simulink model "Channelizer_demo"  (R2023b)
settings: Solver=VariableStepAuto  StartTime=0.0  StopTime=inf  RelTol=1e-3
PostLoadFcn:
  | TT = numerictype(1,16,15);
  | FF = fimath('RoundingMethod','Nearest','OverflowAction','Saturate');
  | mdl = channelizer_init(TT, FF);
  | channelizer = channelizer_model(mdl, TT, FF );
  | Ts = 16*(7/4)/8.75e9;
  | ch_filt_coef = rcosdesign(0.22,4,28,'normal');
  | ch_filt_coef = 28 * ch_filt_coef / sum(ch_filt_coef(:));
  | channelizer_demo_init;
values from neighbouring files (symbols this model uses):
  ch0_en = 0    [channelizer_demo_init.m]    (also in init.m)
  ch0_qam = 0    [channelizer_demo_init.m]    (also in init.m)
  ch0_swp = 0    [channelizer_demo_init.m]    (also in init.m)
  ch10_en = 0    [channelizer_demo_init.m]    (also in init.m)
  ch10_qam = 0    [channelizer_demo_init.m]    (also in init.m)
  ch10_swp = 0    [channelizer_demo_init.m]    (also in init.m)
  ch11_en = 0    [channelizer_demo_init.m]    (also in init.m)
  ch11_qam = 0    [channelizer_demo_init.m]    (also in init.m)
  ch11_swp = 0    [channelizer_demo_init.m]    (also in init.m)
  ch12_en = 0    [channelizer_demo_init.m]    (also in init.m)
  ch12_qam = 0    [channelizer_demo_init.m]    (also in init.m)
  ch12_swp = 0    [channelizer_demo_init.m]    (also in init.m)
  ch13_en = 0    [channelizer_demo_init.m]    (also in init.m)
  ch13_qam = 0    [channelizer_demo_init.m]    (also in init.m)
  ch13_swp = 0    [channelizer_demo_init.m]    (also in init.m)
  ch14_en = 0    [channelizer_demo_init.m]    (also in init.m)
  ch14_qam = 0    [channelizer_demo_init.m]    (also in init.m)
  ch14_swp = 0    [channelizer_demo_init.m]    (also in init.m)
  ch15_en = 0    [channelizer_demo_init.m]    (also in init.m)
  ch15_qam = 0    [channelizer_demo_init.m]    (also in init.m)
  ch15_swp = 0    [channelizer_demo_init.m]    (also in init.m)
  ch1_en = 1    [channelizer_demo_init.m]    (also in init.m)
  ch1_qam = 0    [channelizer_demo_init.m]    (also in init.m)
  ch1_swp = 0    [channelizer_demo_init.m]    (also in init.m)
  ch2_en = 1    [channelizer_demo_init.m]    (also in init.m)
  ch2_qam = 0    [channelizer_demo_init.m]    (also in init.m)
  ch2_swp = 0    [channelizer_demo_init.m]    (also in init.m)
  ch3_en = 0    [channelizer_demo_init.m]    (also in init.m)
  ch3_qam = 0    [channelizer_demo_init.m]    (also in init.m)
  ch3_swp = 0    [channelizer_demo_init.m]    (also in init.m)
  ch4_en = 0    [channelizer_demo_init.m]    (also in init.m)
  ch4_qam = 0    [channelizer_demo_init.m]    (also in init.m)
  ch4_swp = 0    [channelizer_demo_init.m]    (also in init.m)
  ch5_en = 1    [channelizer_demo_init.m]    (also in init.m)
  ch5_qam = 1    [channelizer_demo_init.m]    (also in init.m)
  ch5_swp = 0    [channelizer_demo_init.m]    (also in init.m)
  ch6_en = 1    [channelizer_demo_init.m]    (also in init.m)
  ch6_qam = 1    [channelizer_demo_init.m]    (also in init.m)
  ch6_swp = 0    [channelizer_demo_init.m]    (also in init.m)
  ch7_en = 0    [channelizer_demo_init.m]    (also in init.m)
  ch7_qam = 0    [channelizer_demo_init.m]    (also in init.m)
  ch7_swp = 0    [channelizer_demo_init.m]    (also in init.m)
  ch8_en = 0    [channelizer_demo_init.m]    (also in init.m)
  ch8_qam = 0    [channelizer_demo_init.m]    (also in init.m)
  ch8_swp = 0    [channelizer_demo_init.m]    (also in init.m)
  ch9_en = 0    [channelizer_demo_init.m]    (also in init.m)
  ch9_qam = 0    [channelizer_demo_init.m]    (also in init.m)
  ch9_swp = 0    [channelizer_demo_init.m]    (also in init.m)
  spec1_ch = 1    [channelizer_demo_init.m]    (also in init.m)
  spec2_ch = 2    [channelizer_demo_init.m]    (also in init.m)
  spec3_ch = 5    [channelizer_demo_init.m]    (also in init.m)
  spec4_ch = 6    [channelizer_demo_init.m]    (also in init.m)
  swp_rate0 = 0    [channelizer_demo_init.m]    (also in init.m)
  swp_rate1 = 0    [channelizer_demo_init.m]    (also in init.m)
  swp_rate10 = 0    [channelizer_demo_init.m]    (also in init.m)
  swp_rate11 = 0    [channelizer_demo_init.m]    (also in init.m)
  swp_rate12 = 0    [channelizer_demo_init.m]    (also in init.m)
  swp_rate13 = 0    [channelizer_demo_init.m]    (also in init.m)
  swp_rate14 = 0    [channelizer_demo_init.m]    (also in init.m)
  swp_rate15 = 0    [channelizer_demo_init.m]    (also in init.m)
  swp_rate2 = 0    [channelizer_demo_init.m]    (also in init.m)
  swp_rate3 = 0    [channelizer_demo_init.m]    (also in init.m)
  swp_rate4 = 0    [channelizer_demo_init.m]    (also in init.m)
  swp_rate5 = 0    [channelizer_demo_init.m]    (also in init.m)
  swp_rate6 = 0    [channelizer_demo_init.m]    (also in init.m)
  swp_rate7 = 0    [channelizer_demo_init.m]    (also in init.m)
  swp_rate8 = 0    [channelizer_demo_init.m]    (also in init.m)
  swp_rate9 = 0    [channelizer_demo_init.m]    (also in init.m)
undefined symbols (not defined in the file or in its folder): S, vsva2197, xcvc1902
libraries: aieUtilities x39, aieBasic x34, dspswit3 x16, dspsigops x16, hlsBasic x3, vmcUtilities x1, commchan3 x1
(part 2 of 3)

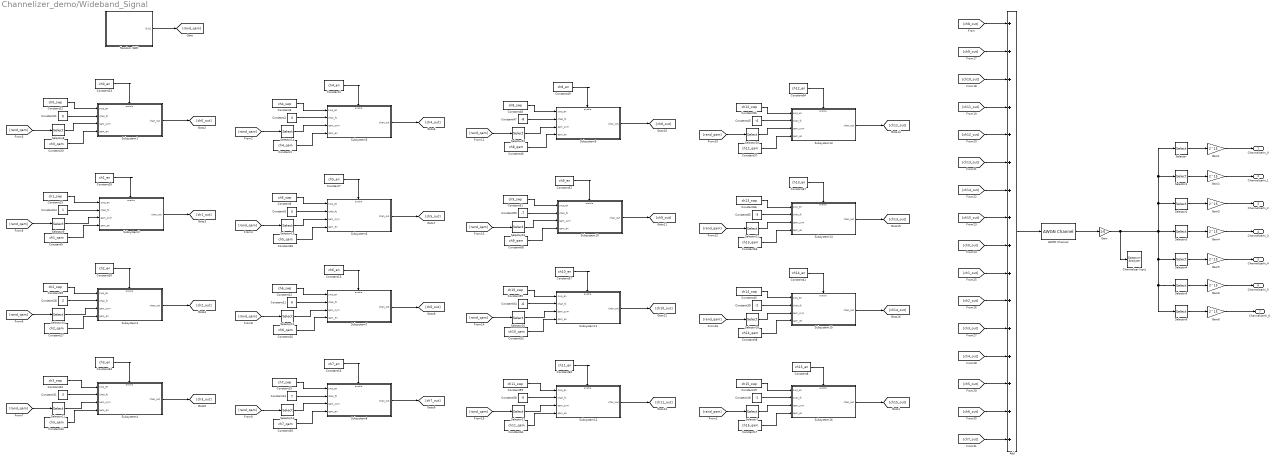
== system Channelizer_demo/Wideband_Signal ==
  AWGN Channel : commchan3/AWGN Channel  LegacyMode=off  NoiseMethod="Signal to noise ratio  (SNR)"  noiseMode="Signal to noise ratio  (SNR)"  EbNo=10  EsNo=10  SNR=20  BitsPerSymbol=1  SignalPower=1  SamplesPerSymbol=1  SymbolPeriod=1  VarianceSource=Input port  Variance=1  RandomStream=Global stream  Seed=67  SimulateUsing=Code generation
  Add : Sum  Inputs=++++++++++++++++
  Channelizer Input : SpectrumAnalyzer  WindowPosition=[1292.000000,660.000000,692.000000,728.000000,]  Visible=on  ScopeFrameLocation=window  SpectrumType=Power density  ViewType=Spectrum and spectrogram  Span=8750000000  StartFrequency=-4375000000  StopFrequency=4375000000  ForgettingFactor=0.4  SpectrumUnits=dBm/Hz  YLimits=[-116.30138229,-48.05166484]  ColorLimits=[-116.30138229,-48.05166484]
  Constant1 : Constant  Value=ch4_qam  SampleTime=-1
  Constant10 : Constant  Value=ch6_qam  SampleTime=-1
  Constant11 : Constant  Value=6  SampleTime=-1
  Constant12 : Constant  Value=ch6_swp  SampleTime=-1
  Constant13 : Constant  Value=ch6_en  SampleTime=-1
  Constant14 : Constant  Value=7  SampleTime=-1
  Constant15 : Constant  Value=ch7_swp  SampleTime=-1
  Constant16 : Constant  Value=ch7_en  SampleTime=-1
  Constant17 : Constant  Value=ch15_qam  SampleTime=-1
  Constant18 : Constant  Value=-1  SampleTime=-1
  Constant19 : Constant  Value=ch15_swp  SampleTime=-1
  Constant2 : Constant  Value=4  SampleTime=-1
  Constant20 : Constant  Value=ch0_qam  SampleTime=-1
  Constant21 : Constant  Value=0  SampleTime=-1
  Constant22 : Constant  Value=ch0_swp  SampleTime=-1
  Constant23 : Constant  Value=ch0_en  SampleTime=-1
  Constant24 : Constant  SampleTime=-1
  Constant25 : Constant  Value=ch1_swp  SampleTime=-1
  Constant26 : Constant  Value=ch1_en  SampleTime=-1
  Constant27 : Constant  Value=ch2_qam  SampleTime=-1
  Constant28 : Constant  Value=2  SampleTime=-1
  Constant29 : Constant  Value=ch2_swp  SampleTime=-1
  Constant3 : Constant  Value=ch4_swp  SampleTime=-1
  Constant30 : Constant  Value=ch2_en  SampleTime=-1
  Constant31 : Constant  Value=3  SampleTime=-1
  Constant32 : Constant  Value=ch3_swp  SampleTime=-1
  Constant33 : Constant  Value=ch3_en  SampleTime=-1
  Constant34 : Constant  Value=ch3_qam  SampleTime=-1
  Constant35 : Constant  Value=ch7_qam  SampleTime=-1
  Constant36 : Constant  Value=ch5_qam  SampleTime=-1
  Constant37 : Constant  Value=ch12_qam  SampleTime=-1
  Constant38 : Constant  Value=ch14_qam  SampleTime=-1
  Constant39 : Constant  Value=-2  SampleTime=-1
  Constant4 : Constant  Value=ch4_en  SampleTime=-1
  Constant40 : Constant  Value=ch14_swp  SampleTime=-1
  Constant41 : Constant  Value=ch14_en  SampleTime=-1
  Constant45 : Constant  Value=-4  SampleTime=-1
  Constant46 : Constant  Value=ch8_qam  SampleTime=-1
  Constant47 : Constant  Value=-8  SampleTime=-1
  Constant48 : Constant  Value=ch8_swp  SampleTime=-1
  Constant49 : Constant  Value=ch8_en  SampleTime=-1
  Constant5 : Constant  Value=5  SampleTime=-1
  Constant50 : Constant  Value=-7  SampleTime=-1
  Constant51 : Constant  Value=ch9_swp  SampleTime=-1
  Constant52 : Constant  Value=ch9_en  SampleTime=-1
  Constant53 : Constant  Value=ch10_qam  SampleTime=-1
  Constant54 : Constant  Value=-6  SampleTime=-1
  Constant55 : Constant  Value=ch10_swp  SampleTime=-1
  Constant56 : Constant  Value=ch12_swp  SampleTime=-1
  Constant57 : Constant  Value=ch10_en  SampleTime=-1
  Constant58 : Constant  Value=-5  SampleTime=-1
  Constant59 : Constant  Value=ch11_swp  SampleTime=-1
  Constant6 : Constant  Value=ch5_swp  SampleTime=-1
  Constant60 : Constant  Value=ch11_en  SampleTime=-1
  Constant61 : Constant  Value=ch11_qam  SampleTime=-1
  Constant63 : Constant  Value=ch13_qam  SampleTime=-1
  Constant64 : Constant  Value=ch12_en  SampleTime=-1
  Constant65 : Constant  Value=-3  SampleTime=-1
  Constant66 : Constant  Value=ch13_swp  SampleTime=-1
  Constant67 : Constant  Value=ch13_en  SampleTime=-1
  Constant68 : Constant  Value=ch9_qam  SampleTime=-1
  Constant7 : Constant  Value=ch5_en  SampleTime=-1
  Constant8 : Constant  Value=ch15_en  SampleTime=-1
  Constant9 : Constant  Value=ch1_qam  SampleTime=-1
  Gain : Gain  Gain=1/6
  Gain{1..6,8} (7 alike) : Gain  Gain=2^15  OutDataTypeStr=int16
  Random QAM : Subsystem
  Selector : Selector  InputPortWidth=28  IndexOptions=Index vector (dialog)  Indices=[14 7 28 21]  OutputSizes=1
  Selector1 : Selector  InputPortWidth=28  IndexOptions=Index vector (dialog)  Indices=[13 6 27 20]  OutputSizes=1
  Selector{8..18,20..23} (15 alike) : Selector  InputPortWidth=16  IndexOptions=Index vector (dialog)  Indices=[9]  OutputSizes=1
  Selector2 : Selector  InputPortWidth=28  IndexOptions=Index vector (dialog)  Indices=[12 5 26 19]  OutputSizes=1
  Selector3 : Selector  InputPortWidth=28  IndexOptions=Index vector (dialog)  Indices=[11 4 25 18]  OutputSizes=1
  Selector4 : Selector  InputPortWidth=28  IndexOptions=Index vector (dialog)  Indices=[10 3 24 17]  OutputSizes=1
  Selector5 : Selector  InputPortWidth=28  IndexOptions=Index vector (dialog)  Indices=[9 2 23 16]  OutputSizes=1
  Selector6 : Selector  InputPortWidth=28  IndexOptions=Index vector (dialog)  Indices=[8 1 22 15]  OutputSizes=1
  Selector7 : Selector  InputPortWidth=16  IndexOptions=Index vector (dialog)  Indices=[8]  OutputSizes=1
  Subsystem1 : Subsystem
  Subsystem10 : Subsystem
  Subsystem11 : Subsystem
  Subsystem12 : Subsystem
  Subsystem13 : Subsystem
  Subsystem14 : Subsystem
  Subsystem15 : Subsystem
  Subsystem16 : Subsystem
  Subsystem2 : Subsystem
  Subsystem3 : Subsystem
  Subsystem4 : Subsystem
  Subsystem5 : Subsystem
  Subsystem6 : Subsystem
  Subsystem7 : Subsystem
  Subsystem8 : Subsystem
  Subsystem9 : Subsystem
  ChannelizerIn_0 : Outport
  ChannelizerIn_1 : Outport  Port=2
  ChannelizerIn_2 : Outport  Port=3
  ChannelizerIn_3 : Outport  Port=4
  ChannelizerIn_4 : Outport  Port=5
  ChannelizerIn_5 : Outport  Port=6
  ChannelizerIn_6 : Outport  Port=7
  wires:
  Add/1 -> AWGN Channel/1
  Constant18/1 -> Subsystem16/2(chan_fc)
  Constant19/1 -> Subsystem16/1(swp_en)
  Constant8/1 -> Subsystem16/Enable
  Constant17/1 -> Subsystem16/4(qam_en)
  Random QAM/1(Out1) -> [rand_qam]
  Selector7/1 -> Subsystem16/3(qam_sym)
  [rand_qam] -> Selector7/1
  Subsystem16/1(chan_out) -> [ch15_out]
  Subsystem1/1(chan_out) -> [ch0_out]
  Constant20/1 -> Subsystem1/4(qam_en)
  Selector8/1 -> Subsystem1/3(qam_sym)
  [rand_qam] -> Selector8/1
  Constant23/1 -> Subsystem1/Enable
  Constant21/1 -> Subsystem1/2(chan_fc)
  Constant22/1 -> Subsystem1/1(swp_en)
  Subsystem2/1(chan_out) -> [ch1_out]
  Selector9/1 -> Subsystem2/3(qam_sym)
  [rand_qam] -> Selector9/1
  Constant26/1 -> Subsystem2/Enable
  Constant24/1 -> Subsystem2/2(chan_fc)
  Constant9/1 -> Subsystem2/4(qam_en)
  Constant25/1 -> Subsystem2/1(swp_en)
  [rand_qam] -> Selector11/1
  Constant28/1 -> Subsystem3/2(chan_fc)
  Constant29/1 -> Subsystem3/1(swp_en)
  Selector11/1 -> Subsystem4/3(qam_sym)
  Constant32/1 -> Subsystem4/1(swp_en)
  Constant30/1 -> Subsystem3/Enable
  [rand_qam] -> Selector10/1
  Selector10/1 -> Subsystem3/3(qam_sym)
  Subsystem4/1(chan_out) -> [ch3_out]
  Constant33/1 -> Subsystem4/Enable
  Constant31/1 -> Subsystem4/2(chan_fc)
  Constant27/1 -> Subsystem3/4(qam_en)
  Subsystem3/1(chan_out) -> [ch2_out]
  Constant34/1 -> Subsystem4/4(qam_en)
  Constant2/1 -> Subsystem5/2(chan_fc)
  [rand_qam] -> Selector15/1
  Constant12/1 -> Subsystem7/1(swp_en)
  Constant15/1 -> Subsystem8/1(swp_en)
  Constant5/1 -> Subsystem6/2(chan_fc)
  Constant35/1 -> Subsystem8/4(qam_en)
  Constant36/1 -> Subsystem6/4(qam_en)
  [rand_qam] -> Selector13/1
  Selector14/1 -> Subsystem5/3(qam_sym)
  Subsystem6/1(chan_out) -> [ch5_out]
  Constant7/1 -> Subsystem6/Enable
  Subsystem8/1(chan_out) -> [ch7_out]
  Subsystem5/1(chan_out) -> [ch4_out]
  Constant4/1 -> Subsystem5/Enable
  Constant16/1 -> Subsystem8/Enable
  Constant1/1 -> Subsystem5/4(qam_en)
  Subsystem7/1(chan_out) -> [ch6_out]
  Constant13/1 -> Subsystem7/Enable
  Constant6/1 -> Subsystem6/1(swp_en)
  [rand_qam] -> Selector14/1
  Selector15/1 -> Subsystem6/3(qam_sym)
  Constant3/1 -> Subsystem5/1(swp_en)
  Selector13/1 -> Subsystem8/3(qam_sym)
  [rand_qam] -> Selector12/1
  Constant14/1 -> Subsystem8/2(chan_fc)
  Subsystem9/1(chan_out) -> [ch8_out]
  Selector20/1 -> Subsystem13/3(qam_sym)
  Constant68/1 -> Subsystem10/4(qam_en)
  Constant47/1 -> Subsystem9/2(chan_fc)
  Constant37/1 -> Subsystem13/4(qam_en)
  Selector16/1 -> Subsystem11/3(qam_sym)
  Constant63/1 -> Subsystem14/4(qam_en)
  Constant56/1 -> Subsystem13/1(swp_en)
  Selector22/1 -> Subsystem9/3(qam_sym)
  [rand_qam] -> Selector21/1
  [rand_qam] -> Selector20/1
  Constant61/1 -> Subsystem12/4(qam_en)
  Constant39/1 -> Subsystem15/2(chan_fc)
  Subsystem14/1(chan_out) -> [ch13_out]
  Constant60/1 -> Subsystem12/Enable
  Constant66/1 -> Subsystem14/1(swp_en)
  Constant51/1 -> Subsystem10/1(swp_en)
  Constant67/1 -> Subsystem14/Enable
  Constant49/1 -> Subsystem9/Enable
  Constant65/1 -> Subsystem14/2(chan_fc)
  Subsystem11/1(chan_out) -> [ch10_out]
  [rand_qam] -> Selector18/1
  Selector23/1 -> Subsystem10/3(qam_sym)
  Constant55/1 -> Subsystem11/1(swp_en)
  Constant59/1 -> Subsystem12/1(swp_en)
  Constant52/1 -> Subsystem10/Enable
  Constant45/1 -> Subsystem13/2(chan_fc)
  Constant40/1 -> Subsystem15/1(swp_en)
  Subsystem10/1(chan_out) -> [ch9_out]
  Subsystem13/1(chan_out) -> [ch12_out]
  Selector18/1 -> Subsystem15/3(qam_sym)
  Constant64/1 -> Subsystem13/Enable
  Selector17/1 -> Subsystem12/3(qam_sym)
  Constant53/1 -> Subsystem11/4(qam_en)
  [rand_qam] -> Selector17/1
  Constant46/1 -> Subsystem9/4(qam_en)
  Selector21/1 -> Subsystem14/3(qam_sym)
  Constant57/1 -> Subsystem11/Enable
  [rand_qam] -> Selector22/1
  Subsystem15/1(chan_out) -> [ch14_out]
  Constant54/1 -> Subsystem11/2(chan_fc)
  Constant41/1 -> Subsystem15/Enable
  Constant48/1 -> Subsystem9/1(swp_en)
  Constant50/1 -> Subsystem10/2(chan_fc)
  [rand_qam] -> Selector16/1
  Constant58/1 -> Subsystem12/2(chan_fc)
  Constant38/1 -> Subsystem15/4(qam_en)
  Subsystem12/1(chan_out) -> [ch11_out]
  [rand_qam] -> Selector23/1
  [ch8_out] -> Add/1
  [ch9_out] -> Add/2
  [ch10_out] -> Add/3
  [ch11_out] -> Add/4
  [ch12_out] -> Add/5
  [ch13_out] -> Add/6
  [ch14_out] -> Add/7
  [ch15_out] -> Add/8
  [ch0_out] -> Add/9
  [ch1_out] -> Add/10
  [ch2_out] -> Add/11
  [ch3_out] -> Add/12
  [ch4_out] -> Add/13
  [ch5_out] -> Add/14
  [ch6_out] -> Add/15
  [ch7_out] -> Add/16
  AWGN Channel/1 -> Gain/1
  Gain/1 -> Selector/1, Selector1/1, Selector2/1, Selector4/1, Selector5/1, Selector6/1, Selector3/1, Channelizer Input/1
  Selector/1 -> Gain1/1
  Selector1/1 -> Gain2/1
  Selector2/1 -> Gain3/1
  Selector3/1 -> Gain4/1
  Selector4/1 -> Gain5/1
  Selector5/1 -> Gain6/1
  Selector6/1 -> Gain8/1
  Gain1/1 -> ChannelizerIn_0/1
  Gain2/1 -> ChannelizerIn_1/1
  Gain3/1 -> ChannelizerIn_2/1
  Gain4/1 -> ChannelizerIn_3/1
  Gain5/1 -> ChannelizerIn_4/1
  Gain6/1 -> ChannelizerIn_5/1
  Gain8/1 -> ChannelizerIn_6/1
  Constant10/1 -> Subsystem7/4(qam_en)
  Selector12/1 -> Subsystem7/3(qam_sym)
  Constant11/1 -> Subsystem7/2(chan_fc)

== system Channelizer_demo/untitledPanel ==
  Slider Switch : SliderSwitchBlock  Tag=HiddenForWebPanel  PanelInfo="{\"addnFilesFolder\":\"\",\"height\":45,\"includeDebugPackages\":false,\"left\":18,\"outputFolder\":\"\",\"panelId\":\"panelId-97556c30-55ab-4b60-93d9-0d2917df0b0a\",\"popoutMode\":\"\",\"standaloneTitle\":\"\",\"top\":18,\"type\":\"panelChild\",\"version\":\"2019b\",\"width\":120,\"zIndex\":1500002}"
      settings: Values={{'Off', 'On'}, [0 1]}
  panelInfo : PanelWebBlock  Tag=HiddenForWebPanel  PanelInfo="{\"addnFilesFolder\":\"\",\"compacted\":false,\"height\":85,\"includeDebugPackages\":false,\"isActiveTab\":true,\"left\":109,\"name\":\"Panel\",\"outputFolder\":\"\",\"panelId\":\"panelId-97556c30-55ab-4b60-93d9-0d2917df0b0a\",\"popoutData\":{\"height\":174,\"left\":2,\"maximized\":false,\"top\":28,\"width\":348},\"popoutMode\":\"windowHidden\",\"standaloneTitle\":\"\",\"tabIndex\":0,\"tabbedSetId\":\"tabbedSet7094157629\",\"top\":87,\"type\":\"panel\",\"version\":\"2019b\",\"visible\":true,\"width\":160,\"zIndex\":1500002}"  PanelSnapshot=<binary blob, 9632 chars, not shown>

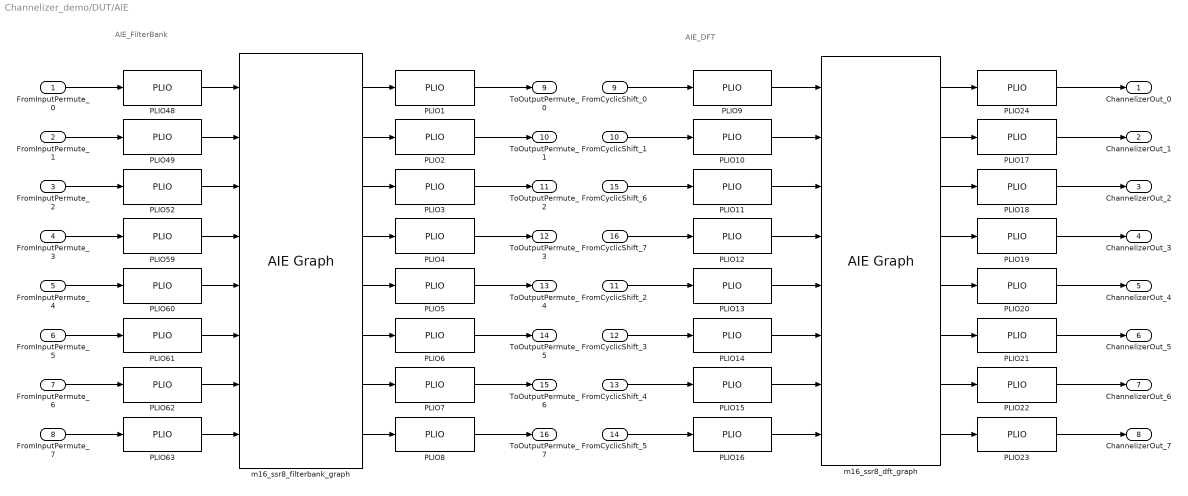
== system Channelizer_demo/DUT/AIE ==
  note: AIE_DFT
  note: AIE_FilterBank
  FromInputPermute_0 : Inport
  FromInputPermute_1 : Inport  Port=2
  FromInputPermute_2 : Inport  Port=3
  FromInputPermute_3 : Inport  Port=4
  FromInputPermute_4 : Inport  Port=5
  FromInputPermute_5 : Inport  Port=6
  FromInputPermute_6 : Inport  Port=7
  FromInputPermute_7 : Inport  Port=8
  FromCyclicShift_0 : Inport  Port=9
  FromCyclicShift_1 : Inport  Port=10
  FromCyclicShift_2 : Inport  Port=11
  FromCyclicShift_3 : Inport  Port=12
  FromCyclicShift_4 : Inport  Port=13
  FromCyclicShift_5 : Inport  Port=14
  FromCyclicShift_6 : Inport  Port=15
  FromCyclicShift_7 : Inport  Port=16
  PLIO{1..24,48..49,52,59..63} (32 alike) : aieBasic/PLIO  PlioWidth=64  PlioFreqSpec=on  PlioFreq=625  ColLocation=0  channel=0  blockJsonConstraints=[]  deprecateConstraints=0
  m16_ssr8_dft_graph : aieBasic/AIE Graph  PortAttributesTable={ 'Input', 'sig_i[0]', 'stream', 'cint16', '', '', ''; 'Input', 'sig_i[1]', 'stream', 'cint16', '', '', ''; 'Input', 'sig_i[6]', 'stream', 'cint16', '', '', ''; 'Input', 'sig_i[7]', 'stream', 'cint16', '', '', ''; 'Input', 'sig_i[2]', 'stream', 'cint16', '', '', ''; 'Input', 'sig_i[3]', 'stream', 'cint16', '', '', ''; 'Input', 'sig_i[4]', 'stream', 'cint16', '', '', ''; 'Input', 'sig_i[5]', 'stream', 'cint16', '', '', ''; 'Output', 'sig_o[0]', 'stream', 'cint16', '', '', '4'; 'Output', 'sig_o[1]', 'stream', 'cint16', '', '', '4'; 'Output', 'sig_o[2]', 'stream', 'cint16', '', '', '4'; 'Output', 'sig_o[3]', 'stream', 'cint16', '', '', '4'; 'Output', 'sig_o[4]', 'stream', 'cint16', '', '', '4'; 'Output', 'sig_o[5]', 'stream', 'cint16', '', '', '4'; 'Output', 'sig_o[6]', 'stream', 'cint16', '', '', '4'; 'Output', 'sig_o[7]', 'stream', 'cint16', '', '', '4' }  PortAttributesEnablement={'off', 'on', 'off', 'off', 'off', 'off', 'off';'off', 'on', 'off', 'off', 'off', 'off', 'off';'off', 'on', 'off', 'off', 'off', 'off', 'off';'off', 'on', 'off', 'off', 'off', 'off', 'off';'off', 'on', 'off', 'off', 'off', 'off', 'off';'off', 'on', 'off', 'off', 'off', 'off', 'off';'off', 'on', 'off', 'off', 'off', 'off', 'off';'off', 'on', 'off', 'off', 'off', 'off', 'off';'off', 'on', 'off', 'off', 'off', 'off', 'on';'off', 'on', 'off', 'off', 'off', 'off', 'on';'off', 'on', 'off', 'off', 'off', 'off', 'on';'off', 'on', 'off', 'off', 'off', 'off', 'on';'off', 'on', 'off', 'off', 'off', 'off', 'on';'off', 'on', 'off', 'off', 'off', 'off', 'on';'off', 'on', 'off', 'off', 'off', 'off', 'on';'off', 'on', 'off', 'off', 'off', 'off', 'on'}  SampleTime=-1  ClassDeclTypeOptions=C[1 1]@t24@class m16_ssr8_dft_graph  ClassDecl=class m16_ssr8_dft_graph  ClassTemplateParams={}  ClassTemplateParamsEnables={}  ClassCtorDeclTypeOptions=C[1 1]@t7@<empty>  ClassCtorDecl=<empty>  ClassCtorParams={}  GraphAllAttrs=|  PortArgDecls={'in stream cint16 in1'; 'in stream cint16 in2'; 'in stream cint16 in3'; 'in stream cint16 in4'; 'in stream cint16 in5'; 'in stream cint16 in6'; 'in stream cint16 in7'; 'in stream cint16 in8'; 'out stream cint16 out1'; 'out stream cint16 out2'; 'out stream cint16 out3'; 'out stream cint16 out4'; 'out stream cint16 out5'; 'out stream cint16 out6'; 'out stream cint16 out7'; 'out stream cint16 out8'}  PortGraphPortNames={'sig_i[0]'; 'sig_i[1]'; 'sig_i[6]'; 'sig_i[7]'; 'sig_i[2]'; 'sig_i[3]'; 'sig_i[4]'; 'sig_i[5]'; 'sig_o[0]'; 'sig_o[1]'; 'sig_o[2]'; 'sig_o[3]'; 'sig_o[4]'; 'sig_o[5]'; 'sig_o[6]'; 'sig_o[7]'}  PortTypes={'stream'; 'stream'; 'stream'; 'stream'; 'stream'; 'stream'; 'stream'; 'stream'; 'stream'; 'stream'; 'stream'; 'stream'; 'stream'; 'stream'; 'stream'; 'stream'}  PortDataTypes={'cint16'; 'cint16'; 'cint16'; 'cint16'; 'cint16'; 'cint16'; 'cint16'; 'cint16'; 'cint16'; 'cint16'; 'cint16'; 'cint16'; 'cint16'; 'cint16'; 'cint16'; 'cint16'}  PortSizes={0.000000000000000000e+00; 0.000000000000000000e+00; 0.000000000000000000e+00; 0.000000000000000000e+00; 0.000000000000000000e+00; 0.000000000000000000e+00; 0.000000000000000000e+00; 0.000000000000000000e+00; 0.000000000000000000e+00; 0.000000000000000000e+00; 0.000000000000000000e+00; 0.000000000000000000e+00; 0.000000000000000000e+00; 0.000000000000000000e+00; 0.000000000000000000e+00; 0.000000000000000000e+00}  PortSynchronicities={'auto'; 'auto'; 'auto'; 'auto'; 'auto'; 'auto'; 'auto'; 'auto'; 'auto'; 'auto'; 'auto'; 'auto'; 'auto'; 'auto'; 'auto'; 'auto'}  PortSignalSizes={0.000000000000000000e+00; 0.000000000000000000e+00; 0.000000000000000000e+00; 0.000000000000000000e+00; 0.000000000000000000e+00; 0.000000000000000000e+00; 0.000000000000000000e+00; 0.000000000000000000e+00; 4.000000000000000000e+00; 4.000000000000000000e+00; 4.000000000000000000e+00; 4.000000000000000000e+00; 4.000000000000000000e+00; 4.000000000000000000e+00; 4.000000000000000000e+00; 4.000000000000000000e+00}  SimLibPath=''  ClassIndex=1  ClassCtorIndex=0  ClassTabVisible=off  FunctionTabVisible=on  DelayDrawLabels=off  GraphFileSelect=Header file (*.h)  GraphHeaderFile=./aie/m16_ssr8_dft_graph.h  GraphClassName=m16_ssr8_dft_graph  GraphName=m16_ssr8_dft_graph  GraphHeaderFiles={'./aie/dft_1xN_widget_graph.h'; './aie/m16_ssr8_dft_graph.h'}  GraphSourceFile=./model_composer_work/xmc_aie_lib/8d40d72d/mygraph.cpp  GraphSearchPaths={'./aie'}  GraphPreProcOptions={}  blockJsonConstraints=[]
      | s[12;12;9;9;19;14;21;23;21;23;24;21;15;17;12;24;26;26;26;27;28;9;21;23;23;23;24;25;14;19;19;29]@FunctionNameDeclFileNamePortNamesPortTypesPortSerializedTypesPortDirectionsPortWindowSizeEnablesPortWindowMarginEnablesPortBufferSizeEnablesPortBufferMarginEnablesPortSynchronicityEnablesPortSignalSizeEnablesPortBufferSizesPortBufferMarginsFunctionDeclFunctionTemplateSpecKindFunctionTemplateParamNamesFunctionTemplateParamKindsFunctionTemplateParamTypesFunctionTemplateParamValuesFunctionTemplateParamEnablesClassDeclClassTemplateSpecKindClassTemplateParamNamesClassTemplateParamKindsClassTemplateParamTypesClassTemplateParamValuesClassTemplateParamEnablesClassCtorDeclsClassCtorParamNamesClassCtorParamTypesClassCtorParamSerializedTypes[1 1]@C[32 1]@nt30@../../aie/m16_ssr8_dft_graph.hC[2 1]@t5@sig_it5@sig_oC[2 1]@t48@std::array< adf::port< adf::direction::in >, 8 >t49@std::array< adf::port< adf::direction::out >, 8 >C[2 1]@t64@{Tstd::array{2{t{Tadf::port{1{t{Sadf::direction::in}}}}}{t{}8}}}t65@{Tstd::array{2{t{Tadf::port{1{t{Sadf::direction::out}}}}}{t{}8}}}C[2 1]@t5@inputt5@inputC[2 1]@l0@l0@C[2 1]@l0@l0@C[2 1]@l0@l0@C[2 1]@l0@l0@C[2 1]@l1@l1@C[2 1]@l0@l0@C[2 1]@nnC[2 1]@nnt139@void m16_ssr8_dft_graph::
      | (std::array< adf::port< adf::direction::in >, 8 > sig_i, std::array< adf::port< adf::direction::out >, 8 > sig_o)ne[0 1]@e[0 1]@e[0 1]@e[0 1]@e[0 1]@t25@class m16_ssr8_dft_graph;t4@nonee[0 1]@e[0 1]@e[0 1]@e[0 1]@e[0 1]@e[0 1]@e[0 1]@e[0 1]@e[0 1]@
  m16_ssr8_filterbank_graph : aieBasic/AIE Graph  PortAttributesTable={ 'Input', 'sig_i[0]', 'stream', 'cint16', '', '', ''; 'Input', 'sig_i[1]', 'stream', 'cint16', '', '', ''; 'Input', 'sig_i[2]', 'stream', 'cint16', '', '', ''; 'Input', 'sig_i[3]', 'stream', 'cint16', '', '', ''; 'Input', 'sig_i[4]', 'stream', 'cint16', '', '', ''; 'Input', 'sig_i[5]', 'stream', 'cint16', '', '', ''; 'Input', 'sig_i[6]', 'stream', 'cint16', '', '', ''; 'Input', 'sig_i[7]', 'stream', 'cint16', '', '', ''; 'Output', 'sig_o[0]', 'stream', 'cint16', '', '', '4'; 'Output', 'sig_o[1]', 'stream', 'cint16', '', '', '4'; 'Output', 'sig_o[2]', 'stream', 'cint16', '', '', '4'; 'Output', 'sig_o[3]', 'stream', 'cint16', '', '', '4'; 'Output', 'sig_o[4]', 'stream', 'cint16', '', '', '4'; 'Output', 'sig_o[5]', 'stream', 'cint16', '', '', '4'; 'Output', 'sig_o[6]', 'stream', 'cint16', '', '', '4'; 'Output', 'sig_o[7]', 'stream', 'cint16', '', '', '4' }  PortAttributesEnablement={'off', 'on', 'off', 'off', 'off', 'off', 'off';'off', 'on', 'off', 'off', 'off', 'off', 'off';'off', 'on', 'off', 'off', 'off', 'off', 'off';'off', 'on', 'off', 'off', 'off', 'off', 'off';'off', 'on', 'off', 'off', 'off', 'off', 'off';'off', 'on', 'off', 'off', 'off', 'off', 'off';'off', 'on', 'off', 'off', 'off', 'off', 'off';'off', 'on', 'off', 'off', 'off', 'off', 'off';'off', 'on', 'off', 'off', 'off', 'off', 'on';'off', 'on', 'off', 'off', 'off', 'off', 'on';'off', 'on', 'off', 'off', 'off', 'off', 'on';'off', 'on', 'off', 'off', 'off', 'off', 'on';'off', 'on', 'off', 'off', 'off', 'off', 'on';'off', 'on', 'off', 'off', 'off', 'off', 'on';'off', 'on', 'off', 'off', 'off', 'off', 'on';'off', 'on', 'off', 'off', 'off', 'off', 'on'}  SampleTime=-1  ClassDeclTypeOptions=C[1 1]@t31@class m16_ssr8_filterbank_graph  ClassDecl=class m16_ssr8_filterbank_graph  ClassTemplateParams={}  ClassTemplateParamsEnables={}  ClassCtorDeclTypeOptions=C[1 1]@t7@<empty>  ClassCtorDecl=<empty>  ClassCtorParams={}  GraphAllAttrs=|  PortArgDecls={'in stream cint16 in1'; 'in stream cint16 in2'; 'in stream cint16 in3'; 'in stream cint16 in4'; 'in stream cint16 in5'; 'in stream cint16 in6'; 'in stream cint16 in7'; 'in stream cint16 in8'; 'out stream cint16 out1'; 'out stream cint16 out2'; 'out stream cint16 out3'; 'out stream cint16 out4'; 'out stream cint16 out5'; 'out stream cint16 out6'; 'out stream cint16 out7'; 'out stream cint16 out8'}  PortGraphPortNames={'sig_i[0]'; 'sig_i[1]'; 'sig_i[2]'; 'sig_i[3]'; 'sig_i[4]'; 'sig_i[5]'; 'sig_i[6]'; 'sig_i[7]'; 'sig_o[0]'; 'sig_o[1]'; 'sig_o[2]'; 'sig_o[3]'; 'sig_o[4]'; 'sig_o[5]'; 'sig_o[6]'; 'sig_o[7]'}  PortTypes={'stream'; 'stream'; 'stream'; 'stream'; 'stream'; 'stream'; 'stream'; 'stream'; 'stream'; 'stream'; 'stream'; 'stream'; 'stream'; 'stream'; 'stream'; 'stream'}  PortDataTypes={'cint16'; 'cint16'; 'cint16'; 'cint16'; 'cint16'; 'cint16'; 'cint16'; 'cint16'; 'cint16'; 'cint16'; 'cint16'; 'cint16'; 'cint16'; 'cint16'; 'cint16'; 'cint16'}  PortSizes={0.000000000000000000e+00; 0.000000000000000000e+00; 0.000000000000000000e+00; 0.000000000000000000e+00; 0.000000000000000000e+00; 0.000000000000000000e+00; 0.000000000000000000e+00; 0.000000000000000000e+00; 0.000000000000000000e+00; 0.000000000000000000e+00; 0.000000000000000000e+00; 0.000000000000000000e+00; 0.000000000000000000e+00; 0.000000000000000000e+00; 0.000000000000000000e+00; 0.000000000000000000e+00}  PortSynchronicities={'auto'; 'auto'; 'auto'; 'auto'; 'auto'; 'auto'; 'auto'; 'auto'; 'auto'; 'auto'; 'auto'; 'auto'; 'auto'; 'auto'; 'auto'; 'auto'}  PortSignalSizes={0.000000000000000000e+00; 0.000000000000000000e+00; 0.000000000000000000e+00; 0.000000000000000000e+00; 0.000000000000000000e+00; 0.000000000000000000e+00; 0.000000000000000000e+00; 0.000000000000000000e+00; 4.000000000000000000e+00; 4.000000000000000000e+00; 4.000000000000000000e+00; 4.000000000000000000e+00; 4.000000000000000000e+00; 4.000000000000000000e+00; 4.000000000000000000e+00; 4.000000000000000000e+00}  SimLibPath=''  ClassIndex=1  ClassCtorIndex=0  ClassTabVisible=off  FunctionTabVisible=on  DelayDrawLabels=off  GraphFileSelect=Header file (*.h)  GraphHeaderFile=./aie/m16_ssr8_filterbank_graph.h  GraphClassName=m16_ssr8_filterbank_graph  GraphName=m16_ssr8_filterbank_graph  GraphHeaderFiles={'./aie/polyphase_fir_graph.h'; './aie/m16_ssr8_filterbank_graph.h'}  GraphSourceFile=./model_composer_work/xmc_aie_lib/fadd8e47/mygraph.cpp  GraphSearchPaths={'./aie'}  GraphPreProcOptions={}  blockJsonConstraints=[]
      | s[12;12;9;9;19;14;21;23;21;23;24;21;15;17;12;24;26;26;26;27;28;9;21;23;23;23;24;25;14;19;19;29]@FunctionNameDeclFileNamePortNamesPortTypesPortSerializedTypesPortDirectionsPortWindowSizeEnablesPortWindowMarginEnablesPortBufferSizeEnablesPortBufferMarginEnablesPortSynchronicityEnablesPortSignalSizeEnablesPortBufferSizesPortBufferMarginsFunctionDeclFunctionTemplateSpecKindFunctionTemplateParamNamesFunctionTemplateParamKindsFunctionTemplateParamTypesFunctionTemplateParamValuesFunctionTemplateParamEnablesClassDeclClassTemplateSpecKindClassTemplateParamNamesClassTemplateParamKindsClassTemplateParamTypesClassTemplateParamValuesClassTemplateParamEnablesClassCtorDeclsClassCtorParamNamesClassCtorParamTypesClassCtorParamSerializedTypes[1 1]@C[32 1]@nt37@../../aie/m16_ssr8_filterbank_graph.hC[2 1]@t5@sig_it5@sig_oC[2 1]@t48@std::array< adf::port< adf::direction::in >, 8 >t49@std::array< adf::port< adf::direction::out >, 8 >C[2 1]@t64@{Tstd::array{2{t{Tadf::port{1{t{Sadf::direction::in}}}}}{t{}8}}}t65@{Tstd::array{2{t{Tadf::port{1{t{Sadf::direction::out}}}}}{t{}8}}}C[2 1]@t5@inputt5@inputC[2 1]@l0@l0@C[2 1]@l0@l0@C[2 1]@l0@l0@C[2 1]@l0@l0@C[2 1]@l1@l1@C[2 1]@l0@l0@C[2 1]@nnC[2 1]@nnt146@void m16_ssr8_filterbank_graph::
      | (std::array< adf::port< adf::direction::in >, 8 > sig_i, std::array< adf::port< adf::direction::out >, 8 > sig_o)ne[0 1]@e[0 1]@e[0 1]@e[0 1]@e[0 1]@t32@class m16_ssr8_filterbank_graph;t4@nonee[0 1]@e[0 1]@e[0 1]@e[0 1]@e[0 1]@e[0 1]@e[0 1]@e[0 1]@e[0 1]@
  ChannelizerOut_0 : Outport
  ChannelizerOut_1 : Outport  Port=2
  ChannelizerOut_2 : Outport  Port=3
  ChannelizerOut_3 : Outport  Port=4
  ChannelizerOut_4 : Outport  Port=5
  ChannelizerOut_5 : Outport  Port=6
  ChannelizerOut_6 : Outport  Port=7
  ChannelizerOut_7 : Outport  Port=8
  ToOutputPermute_0 : Outport  Port=9
  ToOutputPermute_1 : Outport  Port=10
  ToOutputPermute_2 : Outport  Port=11
  ToOutputPermute_3 : Outport  Port=12
  ToOutputPermute_4 : Outport  Port=13
  ToOutputPermute_5 : Outport  Port=14
  ToOutputPermute_6 : Outport  Port=15
  ToOutputPermute_7 : Outport  Port=16
  wires:
  PLIO4/1 -> ToOutputPermute_3/1
  PLIO1/1 -> ToOutputPermute_0/1
  PLIO2/1 -> ToOutputPermute_1/1
  PLIO8/1 -> ToOutputPermute_7/1
  PLIO7/1 -> ToOutputPermute_6/1
  PLIO5/1 -> ToOutputPermute_4/1
  PLIO6/1 -> ToOutputPermute_5/1
  PLIO3/1 -> ToOutputPermute_2/1
  PLIO22/1 -> ChannelizerOut_6/1
  PLIO21/1 -> ChannelizerOut_5/1
  PLIO24/1 -> ChannelizerOut_0/1
  PLIO17/1 -> ChannelizerOut_1/1
  PLIO18/1 -> ChannelizerOut_2/1
  PLIO19/1 -> ChannelizerOut_3/1
  PLIO20/1 -> ChannelizerOut_4/1
  PLIO23/1 -> ChannelizerOut_7/1
  m16_ssr8_filterbank_graph/1 -> PLIO1/1
  m16_ssr8_filterbank_graph/7 -> PLIO7/1
  m16_ssr8_filterbank_graph/6 -> PLIO6/1
  PLIO59/1 -> m16_ssr8_filterbank_graph/4
  PLIO63/1 -> m16_ssr8_filterbank_graph/8
  FromInputPermute_0/1 -> PLIO48/1
  FromInputPermute_4/1 -> PLIO60/1
  PLIO61/1 -> m16_ssr8_filterbank_graph/6
  FromInputPermute_2/1 -> PLIO52/1
  PLIO52/1 -> m16_ssr8_filterbank_graph/3
  FromInputPermute_6/1 -> PLIO62/1
  FromInputPermute_5/1 -> PLIO61/1
  PLIO62/1 -> m16_ssr8_filterbank_graph/7
  FromInputPermute_3/1 -> PLIO59/1
  m16_ssr8_filterbank_graph/5 -> PLIO5/1
  FromInputPermute_7/1 -> PLIO63/1
  PLIO49/1 -> m16_ssr8_filterbank_graph/2
  m16_ssr8_filterbank_graph/8 -> PLIO8/1
  FromInputPermute_1/1 -> PLIO49/1
  PLIO60/1 -> m16_ssr8_filterbank_graph/5
  m16_ssr8_filterbank_graph/3 -> PLIO3/1
  PLIO48/1 -> m16_ssr8_filterbank_graph/1
  m16_ssr8_filterbank_graph/2 -> PLIO2/1
  m16_ssr8_filterbank_graph/4 -> PLIO4/1
  FromCyclicShift_3/1 -> PLIO14/1
  PLIO13/1 -> m16_ssr8_dft_graph/5
  m16_ssr8_dft_graph/8 -> PLIO23/1
  PLIO16/1 -> m16_ssr8_dft_graph/8
  FromCyclicShift_5/1 -> PLIO16/1
  m16_ssr8_dft_graph/1 -> PLIO24/1
  FromCyclicShift_2/1 -> PLIO13/1
  m16_ssr8_dft_graph/3 -> PLIO18/1
  FromCyclicShift_1/1 -> PLIO10/1
  m16_ssr8_dft_graph/6 -> PLIO21/1
  m16_ssr8_dft_graph/5 -> PLIO20/1
  PLIO12/1 -> m16_ssr8_dft_graph/4
  FromCyclicShift_7/1 -> PLIO12/1
  FromCyclicShift_6/1 -> PLIO11/1
  m16_ssr8_dft_graph/2 -> PLIO17/1
  FromCyclicShift_0/1 -> PLIO9/1
  PLIO10/1 -> m16_ssr8_dft_graph/2
  PLIO11/1 -> m16_ssr8_dft_graph/3
  PLIO9/1 -> m16_ssr8_dft_graph/1
  PLIO15/1 -> m16_ssr8_dft_graph/7
  FromCyclicShift_4/1 -> PLIO15/1
  m16_ssr8_dft_graph/4 -> PLIO19/1
  PLIO14/1 -> m16_ssr8_dft_graph/6
  m16_ssr8_dft_graph/7 -> PLIO22/1

== system Channelizer_demo/Wideband_Signal/Random QAM ==
  Constant17 : Constant  Value=3  SampleTime=-1
  Gain7 : Gain  Gain=2
  Gain8 : Gain  Gain=0.5
  Gain9 : Gain  Gain=1/sqrt(10)
  Real-Imag to Complex : RealImagToComplex
  Round : Rounding  Operator=round
  Selector7 : Selector  InputPortWidth=32  IndexOptions=Index vector (dialog)  Indices=1:2:32  OutputSizes=1
  Selector8 : Selector  InputPortWidth=32  IndexOptions=Index vector (dialog)  Indices=2:2:32  OutputSizes=1
  Subtract : Sum  Inputs=+-
  Uniform Random Number : UniformRandomNumber  Maximum=7  Seed=100*(1:32)'  SampleTime=Ts  VectorParams1D=off
  Out1 : Outport
  wires:
  Selector8/1 -> Real-Imag to Complex/2
  Selector7/1 -> Real-Imag to Complex/1
  Gain8/1 -> Round/1
  Subtract/1 -> Gain9/1
  Uniform Random Number/1 -> Gain8/1
  Gain9/1 -> Selector8/1, Selector7/1
  Round/1 -> Gain7/1
  Gain7/1 -> Subtract/1
  Constant17/1 -> Subtract/2
  Real-Imag to Complex/1 -> Out1/1

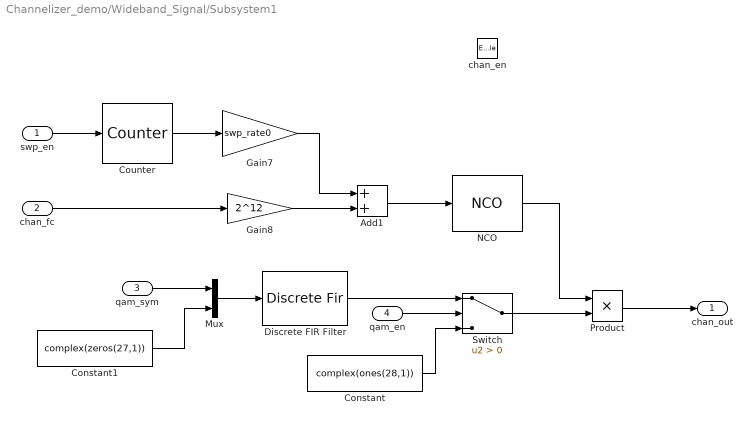
== system Channelizer_demo/Wideband_Signal/Subsystem1 ==
  swp_en : Inport
  chan_fc : Inport  Port=2
  qam_sym : Inport  Port=3
  qam_en : Inport  Port=4
  chan_en : EnablePort
  Add1 : Sum
  Constant : Constant  Value=complex(ones(28,1))  SampleTime=-1
  Constant1 : Constant  Value=complex(zeros(27,1))  SampleTime=-1
  Counter : dspswit3/Counter  Direction=Up  CountEvent=Non-zero sample  CounterSize=User defined  MaxCount=2^31-1  InitialCount=0  Output=Count  HitValue=32  ResetInput=off  SamplesPerFrame=1  Ts=16*(7/4)/8.75e9  CntDtype=int32  HitDtype=Logical
  Discrete FIR Filter : DiscreteFir  Coefficients=ch_filt_coef  InputProcessing=Columns as channels (frame based)
  Gain7 : Gain  Gain=swp_rate0  ParamDataTypeStr=double  OutDataTypeStr=int32  SaturateOnIntegerOverflow=on
  Gain8 : Gain  Gain=2^12  OutDataTypeStr=int32
  Mux : Mux  Inputs=2
  NCO : dspsigops/NCO  AccIncSrc=Input port  AccInc=100  PhaseOffsetSrc=Specify via dialog  PhaseOffset=0  AccumWL=16  HasDither=on  DitherWL=4  PNgeneratorLength=19  HasPhaseQuantizer=on  TableDepth=12  HasOutputPhaseError=off  Formula=Complex exponential  DataType=double  OutputWL=16  OutputFL=14  CompMethod=Table lookup (no interpolation)  SampleTime=1  SamplesPerFrame=28  OutputFrames=off
      settings: LibrarySourceBlock=dspsrcs4/NCO
  Product : Product
  Switch : Switch  Criteria=u2 > Threshold  SaturateOnIntegerOverflow=off  InputSameDT=off
  chan_out : Outport  OutputWhenDisabled=reset  InitialOutput=zeros(28,1)
  wires:
  NCO/1 -> Product/1
  swp_en/1 -> Counter/1
  Add1/1 -> NCO/1
  Product/1 -> chan_out/1
  Gain8/1 -> Add1/2
  Counter/1 -> Gain7/1
  Gain7/1 -> Add1/1
  chan_fc/1 -> Gain8/1
  Switch/1 -> Product/2
  Discrete FIR Filter/1 -> Switch/1
  qam_en/1 -> Switch/2
  Constant/1 -> Switch/3
  Mux/1 -> Discrete FIR Filter/1
  qam_sym/1 -> Mux/1
  Constant1/1 -> Mux/2

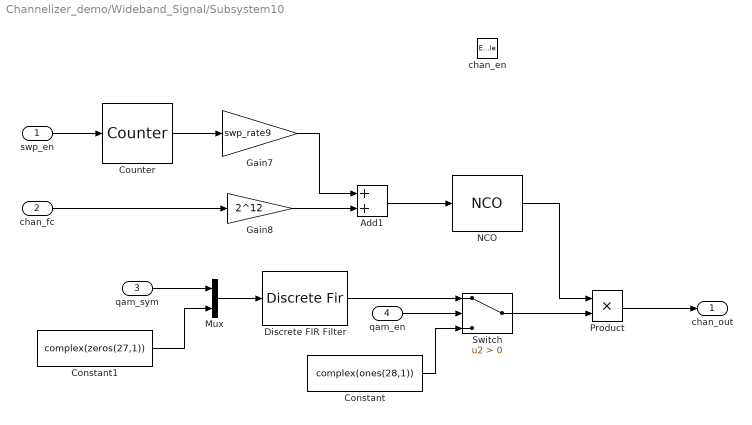
== system Channelizer_demo/Wideband_Signal/Subsystem10 ==
  swp_en : Inport
  chan_fc : Inport  Port=2
  qam_sym : Inport  Port=3
  qam_en : Inport  Port=4
  chan_en : EnablePort
  Add1 : Sum
  Constant : Constant  Value=complex(ones(28,1))  SampleTime=-1
  Constant1 : Constant  Value=complex(zeros(27,1))  SampleTime=-1
  Counter : dspswit3/Counter  Direction=Up  CountEvent=Non-zero sample  CounterSize=User defined  MaxCount=2^31-1  InitialCount=0  Output=Count  HitValue=32  ResetInput=off  SamplesPerFrame=1  Ts=16*(7/4)/8.75e9  CntDtype=int32  HitDtype=Logical
  Discrete FIR Filter : DiscreteFir  Coefficients=ch_filt_coef  InputProcessing=Columns as channels (frame based)
  Gain7 : Gain  Gain=swp_rate9  ParamDataTypeStr=double  OutDataTypeStr=int32  SaturateOnIntegerOverflow=on
  Gain8 : Gain  Gain=2^12  OutDataTypeStr=int32
  Mux : Mux  Inputs=2
  NCO : dspsigops/NCO  AccIncSrc=Input port  AccInc=100  PhaseOffsetSrc=Specify via dialog  PhaseOffset=0  AccumWL=16  HasDither=on  DitherWL=4  PNgeneratorLength=19  HasPhaseQuantizer=on  TableDepth=12  HasOutputPhaseError=off  Formula=Complex exponential  DataType=double  OutputWL=16  OutputFL=14  CompMethod=Table lookup (no interpolation)  SampleTime=1  SamplesPerFrame=28  OutputFrames=off
      settings: LibrarySourceBlock=dspsrcs4/NCO
  Product : Product
  Switch : Switch  Criteria=u2 > Threshold  SaturateOnIntegerOverflow=off  InputSameDT=off
  chan_out : Outport  OutputWhenDisabled=reset  InitialOutput=zeros(28,1)
  wires:
  NCO/1 -> Product/1
  swp_en/1 -> Counter/1
  Add1/1 -> NCO/1
  Product/1 -> chan_out/1
  Gain8/1 -> Add1/2
  Counter/1 -> Gain7/1
  Gain7/1 -> Add1/1
  chan_fc/1 -> Gain8/1
  Switch/1 -> Product/2
  Discrete FIR Filter/1 -> Switch/1
  qam_en/1 -> Switch/2
  Constant/1 -> Switch/3
  Mux/1 -> Discrete FIR Filter/1
  qam_sym/1 -> Mux/1
  Constant1/1 -> Mux/2

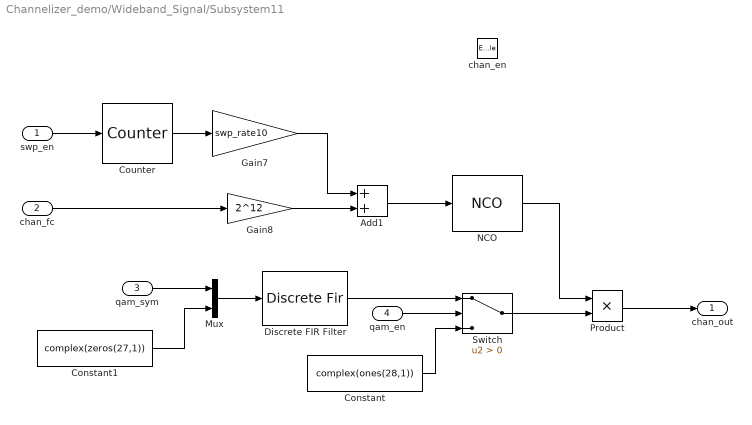
== system Channelizer_demo/Wideband_Signal/Subsystem11 ==
  swp_en : Inport
  chan_fc : Inport  Port=2
  qam_sym : Inport  Port=3
  qam_en : Inport  Port=4
  chan_en : EnablePort
  Add1 : Sum
  Constant : Constant  Value=complex(ones(28,1))  SampleTime=-1
  Constant1 : Constant  Value=complex(zeros(27,1))  SampleTime=-1
  Counter : dspswit3/Counter  Direction=Up  CountEvent=Non-zero sample  CounterSize=User defined  MaxCount=2^31-1  InitialCount=0  Output=Count  HitValue=32  ResetInput=off  SamplesPerFrame=1  Ts=16*(7/4)/8.75e9  CntDtype=int32  HitDtype=Logical
  Discrete FIR Filter : DiscreteFir  Coefficients=ch_filt_coef  InputProcessing=Columns as channels (frame based)
  Gain7 : Gain  Gain=swp_rate10  ParamDataTypeStr=double  OutDataTypeStr=int32  SaturateOnIntegerOverflow=on
  Gain8 : Gain  Gain=2^12  OutDataTypeStr=int32
  Mux : Mux  Inputs=2
  NCO : dspsigops/NCO  AccIncSrc=Input port  AccInc=100  PhaseOffsetSrc=Specify via dialog  PhaseOffset=0  AccumWL=16  HasDither=on  DitherWL=4  PNgeneratorLength=19  HasPhaseQuantizer=on  TableDepth=12  HasOutputPhaseError=off  Formula=Complex exponential  DataType=double  OutputWL=16  OutputFL=14  CompMethod=Table lookup (no interpolation)  SampleTime=1  SamplesPerFrame=28  OutputFrames=off
      settings: LibrarySourceBlock=dspsrcs4/NCO
  Product : Product
  Switch : Switch  Criteria=u2 > Threshold  SaturateOnIntegerOverflow=off  InputSameDT=off
  chan_out : Outport  OutputWhenDisabled=reset  InitialOutput=zeros(28,1)
  wires:
  NCO/1 -> Product/1
  swp_en/1 -> Counter/1
  Add1/1 -> NCO/1
  Product/1 -> chan_out/1
  Gain8/1 -> Add1/2
  Counter/1 -> Gain7/1
  Gain7/1 -> Add1/1
  chan_fc/1 -> Gain8/1
  Switch/1 -> Product/2
  Discrete FIR Filter/1 -> Switch/1
  qam_en/1 -> Switch/2
  Constant/1 -> Switch/3
  Mux/1 -> Discrete FIR Filter/1
  qam_sym/1 -> Mux/1
  Constant1/1 -> Mux/2

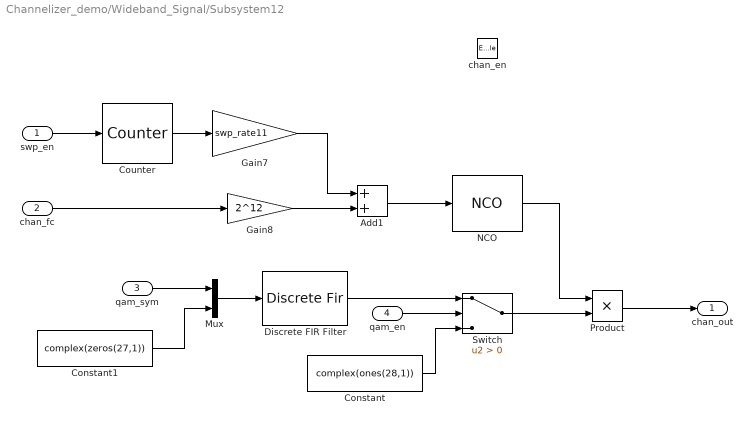
== system Channelizer_demo/Wideband_Signal/Subsystem12 ==
  swp_en : Inport
  chan_fc : Inport  Port=2
  qam_sym : Inport  Port=3
  qam_en : Inport  Port=4
  chan_en : EnablePort
  Add1 : Sum
  Constant : Constant  Value=complex(ones(28,1))  SampleTime=-1
  Constant1 : Constant  Value=complex(zeros(27,1))  SampleTime=-1
  Counter : dspswit3/Counter  Direction=Up  CountEvent=Non-zero sample  CounterSize=User defined  MaxCount=2^31-1  InitialCount=0  Output=Count  HitValue=32  ResetInput=off  SamplesPerFrame=1  Ts=16*(7/4)/8.75e9  CntDtype=int32  HitDtype=Logical
  Discrete FIR Filter : DiscreteFir  Coefficients=ch_filt_coef  InputProcessing=Columns as channels (frame based)
  Gain7 : Gain  Gain=swp_rate11  ParamDataTypeStr=double  OutDataTypeStr=int32  SaturateOnIntegerOverflow=on
  Gain8 : Gain  Gain=2^12  OutDataTypeStr=int32
  Mux : Mux  Inputs=2
  NCO : dspsigops/NCO  AccIncSrc=Input port  AccInc=100  PhaseOffsetSrc=Specify via dialog  PhaseOffset=0  AccumWL=16  HasDither=on  DitherWL=4  PNgeneratorLength=19  HasPhaseQuantizer=on  TableDepth=12  HasOutputPhaseError=off  Formula=Complex exponential  DataType=double  OutputWL=16  OutputFL=14  CompMethod=Table lookup (no interpolation)  SampleTime=1  SamplesPerFrame=28  OutputFrames=off
      settings: LibrarySourceBlock=dspsrcs4/NCO
  Product : Product
  Switch : Switch  Criteria=u2 > Threshold  SaturateOnIntegerOverflow=off  InputSameDT=off
  chan_out : Outport  OutputWhenDisabled=reset  InitialOutput=zeros(28,1)
  wires:
  NCO/1 -> Product/1
  swp_en/1 -> Counter/1
  Add1/1 -> NCO/1
  Product/1 -> chan_out/1
  Gain8/1 -> Add1/2
  Counter/1 -> Gain7/1
  Gain7/1 -> Add1/1
  chan_fc/1 -> Gain8/1
  Switch/1 -> Product/2
  Discrete FIR Filter/1 -> Switch/1
  qam_en/1 -> Switch/2
  Constant/1 -> Switch/3
  Mux/1 -> Discrete FIR Filter/1
  qam_sym/1 -> Mux/1
  Constant1/1 -> Mux/2

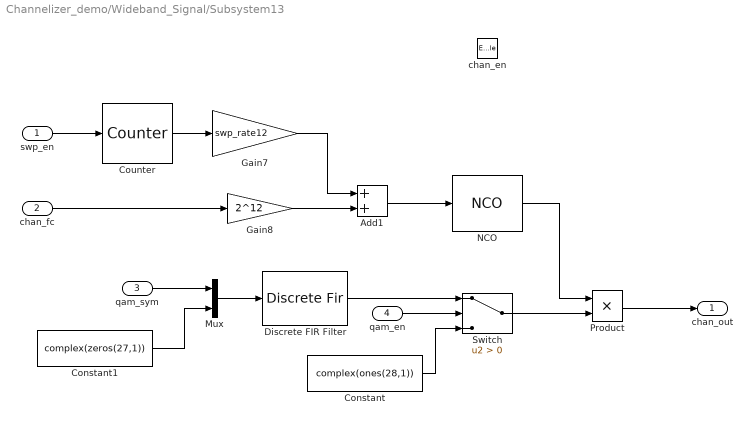
== system Channelizer_demo/Wideband_Signal/Subsystem13 ==
  swp_en : Inport
  chan_fc : Inport  Port=2
  qam_sym : Inport  Port=3
  qam_en : Inport  Port=4
  chan_en : EnablePort
  Add1 : Sum
  Constant : Constant  Value=complex(ones(28,1))  SampleTime=-1
  Constant1 : Constant  Value=complex(zeros(27,1))  SampleTime=-1
  Counter : dspswit3/Counter  Direction=Up  CountEvent=Non-zero sample  CounterSize=User defined  MaxCount=2^31-1  InitialCount=0  Output=Count  HitValue=32  ResetInput=off  SamplesPerFrame=1  Ts=16*(7/4)/8.75e9  CntDtype=int32  HitDtype=Logical
  Discrete FIR Filter : DiscreteFir  Coefficients=ch_filt_coef  InputProcessing=Columns as channels (frame based)
  Gain7 : Gain  Gain=swp_rate12  ParamDataTypeStr=double  OutDataTypeStr=int32  SaturateOnIntegerOverflow=on
  Gain8 : Gain  Gain=2^12  OutDataTypeStr=int32
  Mux : Mux  Inputs=2
  NCO : dspsigops/NCO  AccIncSrc=Input port  AccInc=100  PhaseOffsetSrc=Specify via dialog  PhaseOffset=0  AccumWL=16  HasDither=on  DitherWL=4  PNgeneratorLength=19  HasPhaseQuantizer=on  TableDepth=12  HasOutputPhaseError=off  Formula=Complex exponential  DataType=double  OutputWL=16  OutputFL=14  CompMethod=Table lookup (no interpolation)  SampleTime=1  SamplesPerFrame=28  OutputFrames=off
      settings: LibrarySourceBlock=dspsrcs4/NCO
  Product : Product
  Switch : Switch  Criteria=u2 > Threshold  SaturateOnIntegerOverflow=off  InputSameDT=off
  chan_out : Outport  OutputWhenDisabled=reset  InitialOutput=zeros(28,1)
  wires:
  NCO/1 -> Product/1
  swp_en/1 -> Counter/1
  Add1/1 -> NCO/1
  Product/1 -> chan_out/1
  Gain8/1 -> Add1/2
  Counter/1 -> Gain7/1
  Gain7/1 -> Add1/1
  chan_fc/1 -> Gain8/1
  Switch/1 -> Product/2
  Discrete FIR Filter/1 -> Switch/1
  qam_en/1 -> Switch/2
  Constant/1 -> Switch/3
  Mux/1 -> Discrete FIR Filter/1
  qam_sym/1 -> Mux/1
  Constant1/1 -> Mux/2

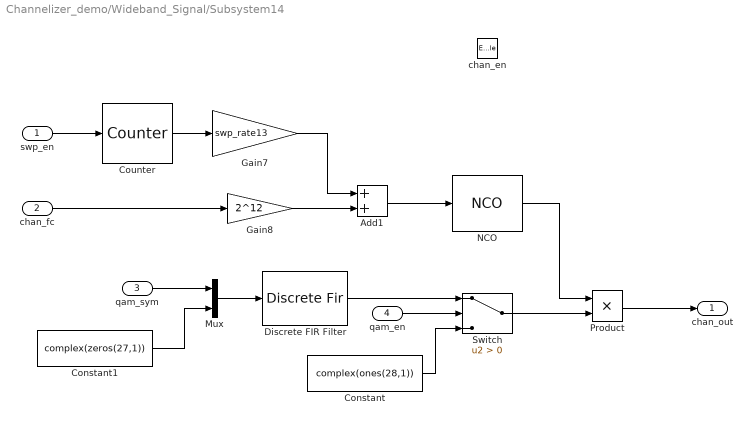
== system Channelizer_demo/Wideband_Signal/Subsystem14 ==
  swp_en : Inport
  chan_fc : Inport  Port=2
  qam_sym : Inport  Port=3
  qam_en : Inport  Port=4
  chan_en : EnablePort
  Add1 : Sum
  Constant : Constant  Value=complex(ones(28,1))  SampleTime=-1
  Constant1 : Constant  Value=complex(zeros(27,1))  SampleTime=-1
  Counter : dspswit3/Counter  Direction=Up  CountEvent=Non-zero sample  CounterSize=User defined  MaxCount=2^31-1  InitialCount=0  Output=Count  HitValue=32  ResetInput=off  SamplesPerFrame=1  Ts=16*(7/4)/8.75e9  CntDtype=int32  HitDtype=Logical
  Discrete FIR Filter : DiscreteFir  Coefficients=ch_filt_coef  InputProcessing=Columns as channels (frame based)
  Gain7 : Gain  Gain=swp_rate13  ParamDataTypeStr=double  OutDataTypeStr=int32  SaturateOnIntegerOverflow=on
  Gain8 : Gain  Gain=2^12  OutDataTypeStr=int32
  Mux : Mux  Inputs=2
  NCO : dspsigops/NCO  AccIncSrc=Input port  AccInc=100  PhaseOffsetSrc=Specify via dialog  PhaseOffset=0  AccumWL=16  HasDither=on  DitherWL=4  PNgeneratorLength=19  HasPhaseQuantizer=on  TableDepth=12  HasOutputPhaseError=off  Formula=Complex exponential  DataType=double  OutputWL=16  OutputFL=14  CompMethod=Table lookup (no interpolation)  SampleTime=1  SamplesPerFrame=28  OutputFrames=off
      settings: LibrarySourceBlock=dspsrcs4/NCO
  Product : Product
  Switch : Switch  Criteria=u2 > Threshold  SaturateOnIntegerOverflow=off  InputSameDT=off
  chan_out : Outport  OutputWhenDisabled=reset  InitialOutput=zeros(28,1)
  wires:
  NCO/1 -> Product/1
  swp_en/1 -> Counter/1
  Add1/1 -> NCO/1
  Product/1 -> chan_out/1
  Gain8/1 -> Add1/2
  Counter/1 -> Gain7/1
  Gain7/1 -> Add1/1
  chan_fc/1 -> Gain8/1
  Switch/1 -> Product/2
  Discrete FIR Filter/1 -> Switch/1
  qam_en/1 -> Switch/2
  Constant/1 -> Switch/3
  Mux/1 -> Discrete FIR Filter/1
  qam_sym/1 -> Mux/1
  Constant1/1 -> Mux/2

== system Channelizer_demo/Wideband_Signal/Subsystem15 ==
  swp_en : Inport
  chan_fc : Inport  Port=2
  qam_sym : Inport  Port=3
  qam_en : Inport  Port=4
  chan_en : EnablePort
  Add1 : Sum
  Constant : Constant  Value=complex(ones(28,1))  SampleTime=-1
  Constant1 : Constant  Value=complex(zeros(27,1))  SampleTime=-1
  Counter : dspswit3/Counter  Direction=Up  CountEvent=Non-zero sample  CounterSize=User defined  MaxCount=2^31-1  InitialCount=0  Output=Count  HitValue=32  ResetInput=off  SamplesPerFrame=1  Ts=16*(7/4)/8.75e9  CntDtype=int32  HitDtype=Logical
  Discrete FIR Filter : DiscreteFir  Coefficients=ch_filt_coef  InputProcessing=Columns as channels (frame based)
  Gain7 : Gain  Gain=swp_rate14  ParamDataTypeStr=double  OutDataTypeStr=int32  SaturateOnIntegerOverflow=on
  Gain8 : Gain  Gain=2^12  OutDataTypeStr=int32
  Mux : Mux  Inputs=2
  NCO : dspsigops/NCO  AccIncSrc=Input port  AccInc=100  PhaseOffsetSrc=Specify via dialog  PhaseOffset=0  AccumWL=16  HasDither=on  DitherWL=4  PNgeneratorLength=19  HasPhaseQuantizer=on  TableDepth=12  HasOutputPhaseError=off  Formula=Complex exponential  DataType=double  OutputWL=16  OutputFL=14  CompMethod=Table lookup (no interpolation)  SampleTime=1  SamplesPerFrame=28  OutputFrames=off
      settings: LibrarySourceBlock=dspsrcs4/NCO
  Product : Product
  Switch : Switch  Criteria=u2 > Threshold  SaturateOnIntegerOverflow=off  InputSameDT=off
  chan_out : Outport  OutputWhenDisabled=reset  InitialOutput=zeros(28,1)
  wires:
  NCO/1 -> Product/1
  swp_en/1 -> Counter/1
  Add1/1 -> NCO/1
  Product/1 -> chan_out/1
  Gain8/1 -> Add1/2
  Counter/1 -> Gain7/1
  Gain7/1 -> Add1/1
  chan_fc/1 -> Gain8/1
  Switch/1 -> Product/2
  Discrete FIR Filter/1 -> Switch/1
  qam_en/1 -> Switch/2
  Constant/1 -> Switch/3
  Mux/1 -> Discrete FIR Filter/1
  qam_sym/1 -> Mux/1
  Constant1/1 -> Mux/2

== system Channelizer_demo/Wideband_Signal/Subsystem16 ==
  swp_en : Inport
  chan_fc : Inport  Port=2
  qam_sym : Inport  Port=3
  qam_en : Inport  Port=4
  chan_en : EnablePort
  Add1 : Sum
  Constant : Constant  Value=complex(ones(28,1))  SampleTime=-1
  Constant1 : Constant  Value=complex(zeros(27,1))  SampleTime=-1
  Counter : dspswit3/Counter  Direction=Up  CountEvent=Non-zero sample  CounterSize=User defined  MaxCount=2^31-1  InitialCount=0  Output=Count  HitValue=32  ResetInput=off  SamplesPerFrame=1  Ts=16*(7/4)/8.75e9  CntDtype=int32  HitDtype=Logical
  Discrete FIR Filter : DiscreteFir  Coefficients=ch_filt_coef  InputProcessing=Columns as channels (frame based)
  Gain7 : Gain  Gain=swp_rate15  ParamDataTypeStr=double  OutDataTypeStr=int32  SaturateOnIntegerOverflow=on
  Gain8 : Gain  Gain=2^12  OutDataTypeStr=int32
  Mux : Mux  Inputs=2
  NCO : dspsigops/NCO  AccIncSrc=Input port  AccInc=100  PhaseOffsetSrc=Specify via dialog  PhaseOffset=0  AccumWL=16  HasDither=on  DitherWL=4  PNgeneratorLength=19  HasPhaseQuantizer=on  TableDepth=12  HasOutputPhaseError=off  Formula=Complex exponential  DataType=double  OutputWL=16  OutputFL=14  CompMethod=Table lookup (no interpolation)  SampleTime=1  SamplesPerFrame=28  OutputFrames=off
      settings: LibrarySourceBlock=dspsrcs4/NCO
  Product : Product
  Switch : Switch  Criteria=u2 > Threshold  SaturateOnIntegerOverflow=off  InputSameDT=off
  chan_out : Outport  OutputWhenDisabled=reset  InitialOutput=zeros(28,1)
  wires:
  NCO/1 -> Product/1
  swp_en/1 -> Counter/1
  Add1/1 -> NCO/1
  Product/1 -> chan_out/1
  Gain8/1 -> Add1/2
  Counter/1 -> Gain7/1
  Gain7/1 -> Add1/1
  chan_fc/1 -> Gain8/1
  Switch/1 -> Product/2
  Discrete FIR Filter/1 -> Switch/1
  qam_en/1 -> Switch/2
  Constant/1 -> Switch/3
  Mux/1 -> Discrete FIR Filter/1
  qam_sym/1 -> Mux/1
  Constant1/1 -> Mux/2
